simulink model "roundabout_onthego_path"  (R2016b)
settings: Solver=FixedStepAuto  StartTime=0.0  StopTime=inf  RelTol=1e-3
undefined symbols (not defined in the file): DiscIntNeverNeededParam, vehicle_name
libraries: simulink x8, SCANeR_API x6
(part 2 of 2)

== matlab function roundabout_onthego_path/MATLAB Function ==
  data: r input; y output [0..1000]; exit input
function y = fcn(r, exit)

 
r_off = 1.5;
lambda = 10; 
degtorad = pi/180;
center_x = 0; 
center_y = 0;
angle = linspace(0, 2*pi, 360); 
x_circle = r*cos(angle) + center_x; 
y_circle = r*sin(angle) + center_y;
circle_start_angle = 10;
qs_x = r_off; qs_y = -30;
p1_x = center_x + (r+r_off)*cos((lambda-90)*degtorad); 
p1_y = center_y + (r+r_off)*sin((lambda-90)*degtorad);
p2_x = center_x + (r)*cos(-lambda*degtorad);
p2_y = center_y + (r)*sin(-lambda*degtorad);

npts = 8 ;

cl1_theta0 = 90*degtorad; cl1_theta1 = 10*degtorad;
cl2_theta0 = 10*degtorad; cl2_theta1 = 30*degtorad; 

[k1,dk1,L1] = buildClothoid(qs_x, qs_y, cl1_theta0, p1_x, p1_y, cl1_theta1);

XY1 = pointsOnClothoid(qs_x, qs_y, cl1_theta0, k1, dk1, L1, npts) ;
XY4 = zeros(size(XY1,1), size(XY1,2)); XY6 = zeros(size(XY1,1), size(XY1,2));
XY8 = zeros(size(XY1,1), size(XY1,2)); XY10 = zeros(size(XY1,1), size(XY1,2));
XY6(1,:) = XY1(1,:); XY6(2,:)= -XY1(2,:);

XY8(1,:) = XY1(2,:); XY8(2,:)=XY1(1,:);

XY10(1,:) = -XY1(1,:); XY10(2,:)=XY1(2,:);

XY4(1,:) = -XY8(1,:); XY4(2,:) = -XY8(2,:);


%---- sequentialize ----------- %


XY4(1,:) = XY4(1,end:-1:1); XY4(2,:) = XY4(2,end:-1:1);

XY6(1,:) = XY6(1,end:-1:1); XY6(2,:) = XY6(2,end:-1:1);

XY8(1,:) = XY8(1,end:-1:1); XY8(2,:) = XY8(2,end:-1:1);

XY10(1,:) = XY10(1,end:-1:1); XY10(2,:) = XY10(2,end:-1:1);



start_deg = 10; deg_len = (90*exit)-(2*start_deg); npts_arc = (deg_len - (exit*20)); step_size = (deg_len/npts_arc); 
arc1_x = zeros(1,npts_arc);
arc1_y = zeros(1,npts_arc);
for i = 1:npts_arc
    ang = start_deg + i*step_size;
    arc1_x(i) = center_x + (r+r_off)*cos((ang-90)*degtorad);
    arc1_y(i) = center_y + (r+r_off)*sin((ang-90)*degtorad);
end


if exit == 1
    comb_x = [XY1(1,:) arc1_x(1,:) XY4(1,:)];
    comb_y = [XY1(2,:) arc1_y(1,:) XY4(2,:)];
end
if exit == 2
    comb_x = [XY1(1,:) arc1_x(1,:) XY6(1,:)];
    comb_y = [XY1(2,:) arc1_y(1,:) XY6(2,:)];
end
if exit == 3
    comb_x = [XY1(1,:) arc1_x(1,:) XY8(1,:)];
    comb_y = [XY1(2,:) arc1_y(1,:) XY8(2,:)];
end
if exit == 4
    comb_x = [XY1(1,:) arc1_x(1,:) XY10(1,:)];
    comb_y = [XY1(2,:) arc1_y(1,:) XY10(2,:)];
end
plot(comb_x, comb_y);

y = [comb_x', comb_y'];
% y = comb_x; 
end

function [ k, dk, L, iter, varargout ] = buildClothoid( x0, y0, theta0, x1, y1, theta1 )

  dx  = x1 - x0 ;
  dy  = y1 - y0 ;
  r   = sqrt( dx^2 + dy^2 ) ;
  phi = atan2( dy, dx ) ;

  phi0  = normalizeAngle(theta0 - phi) ;
  phi1  = normalizeAngle(theta1 - phi) ;
  delta = phi1 - phi0 ;

  % initial point
  Aguess = guessA( phi0, phi1 ) ;

  % Newton iteration
  [A,iter] = findA( Aguess, delta, phi0, 1e-12 ) ;

  % final operation
  [h,g] = GeneralizedFresnelCS( 1, 2*A, delta-A, phi0 ) ;
  L = r/h ;

  if L > 0
    k  = (delta - A)/L ;
    dk = 2*A/L^2 ;
  else
    error('negative length') ;
  end

  if nargout == 10

    [X,Y] = GeneralizedFresnelCS( 3, 2*A, delta-A, theta0 ) ;
    
    if true
      alpha = X(1)*X(2) + Y(1)*Y(2) ;
      beta  = X(1)*X(3) + Y(1)*Y(3) ;
      gamma = X(1)^2+Y(1)^2 ;
      tx    = X(2)-X(3) ;
      ty    = Y(2)-Y(3) ;
      txy   = L*(X(2)*Y(3)-X(3)*Y(2)) ;
      omega = L*(Y(1)*tx-X(1)*ty) - txy ;
      delta = X(1)*tx + Y(1)*ty ;

      L_1  = omega/delta ; % L_0
      L_2  = txy/delta ; % L_1

      delta = delta * L ;
      k_1  = (beta-gamma-k*omega)/delta ; % k_0
      k_2  = -(beta+k*txy)/delta ; % k_1

      delta = delta * L/2 ;
      dk_1 = (gamma-alpha-dk*omega*L)/delta ; % dk_0    
      dk_2 = (alpha-dk*txy*L)/delta ; % dk_1
    else
      dkL = dk*L ;
      M = [ X(1) - L*(dkL*Y(3)+k*Y(2)), -L*Y(2), -L*Y(3) ; ...
            Y(1) + L*(dkL*X(3)+k*X(2)),  L*X(2),  L*X(3) ; ...
            dkL+k,                            1,       1 ] ;
      tmp = M\[L*Y(1);-L*X(1);-1] ;
      L_1  = tmp(1) ;
      k_1  = tmp(2)/L ;
      dk_1 = 2*tmp(3)/L^2 ;
      tmp = M\[0;0;1] ;
      L_2  = tmp(1) ;
      k_2  = tmp(2)/L ;
      dk_2 = 2*tmp(3)/L^2 ;
    end
    
    varargout{1} = k_1 ; % k_0
    varargout{2} = dk_1 ; % dk_0
    varargout{3} = L_1 ; % L_0
    
    varargout{4} = k_2 ; % k_1
    varargout{5} = dk_2 ; % dk_1
    varargout{6} = L_2 ; % L_1

  elseif nargout > 4
    error('expected <= 4 or 10 output argument') ;
  end 
  
end

%=========================================================================%
%  normalizeAngle:  normalize angle in the range [-pi,pi]                 %
%=========================================================================%
function phi = normalizeAngle( phi_in )
  phi = phi_in ;
  while ( phi > pi )
    phi = phi - 2*pi ;
  end
  while ( phi < -pi )
    phi = phi + 2*pi ;
  end
end

%=========================================================================%
%  findA:  Find a zero of function g(A) defined as                        %
%  g(A) = \int_0^1 \sin( A*t^2+(delta-A)*t+phi0 ) dt                      %
%                                                                         %
%  USAGE:  A = findA( Aguess, delta, phi0, tol );                         %
%                                                                         %
%  Given an initial guess Aguess find the closest zero of equation g(A)   %
%                                                                         %
%  On input:                                                              %
%    Aguess      = initial guess.                                         %
%    delta, phi0 = Angles used in the clothoid fitting problem.           %
%    tol         = Tolerance for stopping criterium of Newton iteration.  %
%                                                                         %
%  On output:                                                             %
%    A           = the zero of function g(A) closest to Aguess.           %
%    iter        = iteration performed                                    %
%                                                                         %
%=========================================================================%
function [A,iter] = findA( Aguess, delta, phi0, tol )
  A = Aguess ;
  for iter=1:100
    [intC,intS] = GeneralizedFresnelCS( 3, 2*A, delta-A, phi0 ) ;
    f  = intS(1) ;
    df = intC(3)-intC(2) ;
    A  = A - f/df ;
    if abs(f) < tol
      break ;
    end
  end
  if abs(f) > tol*10
    fprintf( 1, 'Newton iteration fails, f = %g\n', f ) ;
    fprintf( 1, 'Aguess = %g, A = %g, delta = %g , phi0 = %g\n', Aguess, A, delta, phi0 ) ;
  end
end

%=========================================================================%
%  guessA:  Find guess for zeros of function g(A)                         %
%                                                                         %
%  USAGE:  A = guessA( phi0, phi1 );                                      %
%                                                                         %
%  On input:                                                              %
%       phi0, phi1 = Angles used in the clothoid fitting problem.         %
%                                                                         %
%  On output:                                                             %
%       A = an approximate zero of function g(A).                         %
%                                                                         %
%=========================================================================%
function A = guessA( phi0, phi1 )
  CF = [ 2.989696028701907, ...
         0.716228953608281, ...
        -0.458969738821509, ...
        -0.502821153340377, ...
         0.261062141752652, ...
        -0.045854475238709 ] ;
  X  = phi0/pi ;
  Y  = phi1/pi ;
  xy = X*Y ;
  A  = (phi0+phi1) * ( CF(1) + xy * ( CF(2) + xy * CF(3) ) + ...
                       (CF(4) + xy * CF(5)) * (X^2+Y^2) + ...
                        CF(6) * (X^4+Y^4) ) ;
end

function varargout = pointsOnClothoid( varargin )
  
  if nargin == 2
    if isstruct(varargin{1})
      x0     = varargin{1}.x0 ;
      y0     = varargin{1}.y0 ;
      theta0 = varargin{1}.theta0 ;
      kappa  = varargin{1}.kappa ;
      dkappa = varargin{1}.dkappa ;
      L      = varargin{1}.L ;
      npts   = varargin{2} ;
      tvec   = [0:L/(npts-1):L] ;
    else
      error('expexted struct as first arument') ;
    end
  elseif nargin == 6 || nargin == 7
    x0     = varargin{1} ;
    y0     = varargin{2} ;
    theta0 = varargin{3} ;
    kappa  = varargin{4} ;
    dkappa = varargin{5} ;
    L      = varargin{6} ;
    if nargin == 7
      npts = varargin{7} ;
      tvec = [0:L/(npts-1):L] ;
    else
      tvec = L ;
    end
  else
    error('expexted 2,6 or 7 input arguments') ;
  end
  
  X = [] ;
  Y = [] ;
  for t=tvec(1,1):tvec(1,end)
    [C,S] = GeneralizedFresnelCS( 1, dkappa*t^2, kappa*t, theta0 ) ;
    X = [ X x0 + t*C ] ;
    Y = [ Y y0 + t*S ] ;
  end
  if nargout > 1
    varargout{1} = X ;
    varargout{2} = Y ;
  else
    varargout{1} = [X ; Y] ;
  end
end

function [X,Y] = GeneralizedFresnelCS( nk, a, b, c )

  epsi = 1e-2 ; % best thresold

  if abs(a) < epsi % case `a` small
    [X,Y] = evalXYaSmall( nk, a, b, 3 ) ;
  else
    [X,Y] = evalXYaLarge( nk, a, b ) ;
  end

  cc = cos(c) ;
  ss = sin(c) ;

  for k=1:nk
    xx = X(k) ;
    yy = Y(k) ;
    X(k) = xx*cc-yy*ss ;
    Y(k) = xx*ss+yy*cc ;
  end

end
%
%
%
function [C,S] = FresnelCSk( nk, t )
  C = zeros(nk,1) ;
  S = zeros(nk,1) ;
  [C(1),S(1)] = FresnelCS(t) ;
  if nk > 1
    tt   = pi/2*t^2 ;
    ss   = sin(tt) ;
    cc   = cos(tt) ;
    C(2) = ss/pi ;
    S(2) = (1-cc)/pi ;
    if nk > 2
      C(3) = (t*ss-S(1))/pi ;
      S(3) = (C(1)-t*cc)/pi ;
    end
  end
end
%
%
%
function [X,Y] = evalXYaLarge( nk, a, b )
  X       = zeros(nk,1) ;
  Y       = zeros(nk,1) ;
  s       = sign(a) ;
  z       = sqrt(abs(a)/pi) ;
  ell     = s*b/sqrt(abs(a)*pi) ;
  g       = -0.5*s*b^2/abs(a) ;
  [Cl,Sl] = FresnelCSk(nk,ell) ;
  [Cz,Sz] = FresnelCSk(nk,ell+z) ;
  dC      = Cz - Cl ;
  dS      = Sz - Sl ;
  cg      = cos(g)/z ;
  sg      = sin(g)/z ;
  X(1)    = cg * dC(1) - s * sg * dS(1) ;
  Y(1)    = sg * dC(1) + s * cg * dS(1) ;
  if nk > 1
    cg   = cg/z ;
    sg   = sg/z ;
    DC   = dC(2)-ell*dC(1);
    DS   = dS(2)-ell*dS(1);
    X(2) = cg * DC - s * sg * DS ;
    Y(2) = sg * DC + s * cg * DS ;
    if nk > 2
      cg   = cg/z ;
      sg   = sg/z ;
      DC   = dC(3)+ell*(ell*dC(1)-2*dC(2)) ;
      DS   = dS(3)+ell*(ell*dS(1)-2*dS(2)) ;
      X(3) = cg * DC - s * sg * DS ;
      Y(3) = sg * DC + s * cg * DS ;
    end
  end
end
%
%
%
function res = rLommel_MATLAB(mu, nu, z)
  a   = mu-nu+1 ;
  b   = mu+nu+1 ;
  res = eval(hypergeom(1,[a/2+1,b/2+1],-z^2/4)/(a*b)) ;
end
%
%
%
function res = rLommel(mu,nu,b)
  tmp = 1/((mu+nu+1)*(mu-nu+1)) ;
  res = tmp ;
  for n=1:100
    tmp = tmp * (-b/(2*n+mu-nu+1)) * (b/(2*n+mu+nu+1)) ;
    res = res + tmp ;
    if abs(tmp) < abs(res) * 1e-50
      break ;
    end;
  end
end
%
%
%
function [X,Y] = evalXYazero( nk, b )
  X  = zeros(nk,1) ;
  Y  = zeros(nk,1) ;
  sb = sin(b);
  cb = cos(b);
  b2 = b*b ;
  if abs(b) < 1e-3
    X(1) = 1-(b2/6)*(1-(b2/20)*(1-(b2/42))) ;
    Y(1) = (b/2)*(1-(b2/12)*(1-(b2/30))) ;
  else
    X(1) = sb/b ;
    Y(1) = (1-cb)/b ;
  end
  % use recurrence in the stable part
  m = min( [ max([1,floor(2*b)]), nk] ) ;
  for k=1:m-1
    X(k+1) = (sb-k*Y(k))/b ;
    Y(k+1) = (k*X(k)-cb)/b ;
  end
  % use Lommel for the unstable part
  if m < nk
    A   = b*sb ;
    D   = sb-b*cb ;
    B   = b*D ;
    C   = -b2*sb ;
    rLa = rLommel(m+1/2,3/2,b) ;
    rLd = rLommel(m+1/2,1/2,b) ;
    for k=m:nk-1
      rLb    = rLommel(k+3/2,1/2,b) ;
      rLc    = rLommel(k+3/2,3/2,b) ;
      X(k+1) = ( k*A*rLa + B*rLb + cb )/(1+k) ;
      Y(k+1) = ( C*rLc + sb ) / (2+k) + D*rLd ;
      rLa = rLc ;
      rLd = rLb ;
    end
  end
end
%
%
%
function [X,Y] = evalXYaSmall( nk, a, b, p )
  [X0,Y0] = evalXYazero( nk + 4*p + 2, b ) ;

  X    = zeros(nk,1) ;
  Y    = zeros(nk,1) ;
  tmpX = zeros(p+1,1) ;
  tmpY = zeros(p+1,1) ;

  for j=1:nk
    tmpX(1) = X0(j)-(a/2)*Y0(j+2) ;
    tmpY(1) = Y0(j)+(a/2)*X0(j+2) ;
    t  = 1 ;
    aa = -(a/2)^2 ;
    for n=1:p
      ii = 4*n+j ;
      t  = t*(aa/(2*n*(2*n-1))) ;
      bf = a/(4*n+2) ;
      tmpX(1+n) = t*(X0(ii)-bf*Y0(ii+2)) ;
      tmpY(1+n) = t*(Y0(ii)+bf*X0(ii+2)) ;
    end
    X(j) = sum(tmpX) ;
    Y(j) = sum(tmpY) ;
  end
end

function [FresnelC,FresnelS] = FresnelCS(y)
%******************************************************************************
% FresnelCS:  Compute Fresnel sine and cosine integrals                       %
%                                                                             %
% USAGE: [FresnelC,FresnelS] = FresnelCS(y) ;                                 %
%                                                                             %
%  Fresnel integral are defined as:                                           %
%                                                                             %
%  C(y) = \int_0^y cos( (pi/2)*t^2 ) dt                                       %
%  S(y) = \int_0^y sin( (pi/2)*t^2 ) dt                                       %
%                                                                             %
% The algorithm is described in:                                              %
%   Atlas for computing mathematical functions : an illustrated guide for     %
%   practitioners, with programs in C and Mathematica / William J. Thompson.  %
%   New York : Wiley, c1997.                                                  %
%                                                                             %
% The cose is a sligly modification of original code developed by             %
% Venkata Sivakanth Telasula (sivakanth.telasula@gmail.com)                   %
%                                                                             %
% On input:                                                                   %
%                                                                             %
%       y = argument of the function C(y) and S(y), it may be a vector        %
%                                                                             %
% On output:                                                                  %
%                                                                             %
%       FresnelC = The value(s) of C(y)                                       %
%       FresnelS = The value(s) of S(y)                                       %
%                                                                             %
%******************************************************************************

  fn = [ 0.49999988085884732562,   ...
         1.3511177791210715095,    ...
         1.3175407836168659241,    ...
         1.1861149300293854992,    ...
         0.7709627298888346769,    ...
         0.4173874338787963957,    ...
         0.19044202705272903923,   ...
         0.06655998896627697537,   ...
         0.022789258616785717418,  ...
         0.0040116689358507943804, ...
         0.0012192036851249883877 ] ;
  
  fd = [ 1.0,                      ...
         2.7022305772400260215,    ...
         4.2059268151438492767,    ...
         4.5221882840107715516,    ...
         3.7240352281630359588,    ...
         2.4589286254678152943,    ...
         1.3125491629443702962,    ...
         0.5997685720120932908,    ...
         0.20907680750378849485,   ...
         0.07159621634657901433,   ...
         0.012602969513793714191,  ...
         0.0038302423512931250065 ] ;
  
  gn = [ 0.50000014392706344801,    ...
         0.032346434925349128728,   ...
         0.17619325157863254363,    ...
         0.038606273170706486252,   ...
         0.023693692309257725361,   ...
         0.007092018516845033662,   ...
         0.0012492123212412087428,  ...
         0.00044023040894778468486, ...
        -8.80266827476172521e-6,    ...
        -1.4033554916580018648e-8,  ...
        2.3509221782155474353e-10 ] ;
  
  gd  = [ 1.0,                      ...
          2.0646987497019598937,    ...
          2.9109311766948031235,    ...
          2.6561936751333032911,    ...
          2.0195563983177268073,    ...
          1.1167891129189363902,    ...
          0.57267874755973172715,   ...
          0.19408481169593070798,   ...
          0.07634808341431248904,   ...
          0.011573247407207865977,  ...
          0.0044099273693067311209, ...
         -0.00009070958410429993314 ] ;

  FresnelC = zeros(size(y));
  FresnelS = zeros(size(y));
  
  for j = 1:length(y)
    x = abs(y(j)) ;
    if x < 1.0
      t = -((pi/2)*x.^2).^2;
      % Cosine integral series
      twofn   = 0.0 ;
      fact    = 1.0 ;
      denterm = 1.0 ;
      numterm = 1.0 ;
      sum     = 1.0 ;
      ratio   = 10.0 ; 
 
      while ratio > eps
        twofn   = twofn + 2.0;
        fact    = fact*twofn*(twofn-1.0);
        denterm = denterm + 4.0;
        numterm = numterm*t;
        term    = numterm/(fact*denterm);
        sum     = sum+term;
        ratio   = abs(term/sum);
      end

      FresnelC(j) = x*sum;
 
      % Sine integral series
      twofn   = 1.0 ;
      fact    = 1.0 ;
      denterm = 3.0 ;
      numterm = 1.0 ;
      sum     = 1.0/3.0 ;
      ratio   = 10.0 ;
 
      while ratio > eps
        twofn   = twofn+2.0;
        fact    = fact*twofn*(twofn-1.0);
        denterm = denterm+4.0;
        numterm = numterm*t;
        term    = numterm/(fact*denterm);
        sum     = sum+term;
        ratio   = abs(term/sum);
      end
 
      FresnelS(j) = (pi/2)*sum.*x.^3;

    elseif x < 6.0

      % Rational approximation for f
      sumn = 0.0 ;
      sumd = fd(12) ;
      for k=11:-1:1
        sumn = fn(k)+x*sumn ;
        sumd = fd(k)+x*sumd ;
      end
      f = sumn/sumd;
      % Rational approximation for  g
      sumn = 0.0 ;
      sumd = gd(12) ;
      for k=11:-1:1
        sumn = gn(k)+x*sumn;
        sumd = gd(k)+x*sumd;
      end
      g    = sumn/sumd;
      U    = (pi/2)*x.^2 ;
      SinU = sin(U);
      CosU = cos(U);
      FresnelC(j) = 0.5+f*SinU-g*CosU;
      FresnelS(j) = 0.5-f*CosU-g*SinU;
    else
      % x >= 6; asymptotic expansions for  f  and  g
      t = -(pi*x.^2)^(-2.0) ;
      % Expansion for  f
      numterm = -1.0 ;
      term    =  1.0 ;
      sum     =  1.0 ;
      oldterm =  1.0 ;
      ratio   = 10.0 ;
      eps10   = 0.1*eps;

      while ratio > eps10
        numterm = numterm+4.0;
        term    = term*numterm*(numterm-2.0)*t;
        sum     = sum + term;
        absterm = abs(term);
        ratio   = abs(term/sum);
        if oldterm < absterm
          disp('\n\n !!In FresnelCS f not converged to eps');
          ratio = eps10;
        end
        oldterm = absterm;
      end

      f = sum/(pi*x);
      % Expansion for  g
      numterm = -1.0 ;
      term    =  1.0 ;
      sum     =  1.0 ;
      oldterm =  1.0 ; 
      ratio   = 10.0 ;
      eps10   = 0.1*eps ;

      while ratio > eps10
        numterm = numterm+ 4.0;
        term    = term*numterm*(numterm+2.0)*t;
        sum     = sum+term;
        absterm = abs(term);
        ratio   = abs(term/sum);
        if oldterm < absterm
          disp('\n\n!!In FresnelCS g not converged to eps');
          ratio = eps10;
        end
        oldterm = absterm;
      end
      g    = sum/((pi*x)^2*x) ;
      U    = (pi/2)*x.^2 ;
      SinU = sin(U);
      CosU = cos(U);
      FresnelC(j) = 0.5+f*SinU-g*CosU;
      FresnelS(j) = 0.5-f*CosU-g*SinU;
    end
    if y(j) < 0
      FresnelC(j) = -FresnelC(j) ;
      FresnelS(j) = -FresnelS(j) ;
    end
  end
end
% EOF

== stateflow chart roundabout_onthego_path/Subsystem/Chart1 ==
  state Speed_Control/
    state Control_Off/
      accel = 0;
      brake = 0;
      int_epsilon = 0;
      Gear=3;
    state Controller/
      limit_accel = 1/kp_acc;
      limit_brake = 1/kp_brk;
      state normal_regulation/
        state normal_accel/
          control_state = 2;
          accel = -kp_acc*epsilon - ki_acc*int_epsilon;
          brake = 0;
          Gear_d = Gear;
        state normal_brake/
          control_state = 1;
          brake = kp_brk*epsilon + ki_brk*int_epsilon;
          accel = 0;
          Gear_d = Gear;
        (junction 58) -> (junction 59) [order 1] : [epsilon <= tolerance]
        (junction 58) -> (junction 57) [order 2]
        (junction 59) -> Speed_Control.Controller.normal_regulation.normal_accel [order 1] : [abs(epsilon) < limit_accel & control_state == 2]
            | {int_epsilon = int_epsilon + step_size*epsilon;}
        (junction 59) -> Speed_Control.Controller.normal_regulation.normal_accel [order 2] : {int_epsilon = 0;}
        (junction 57) -> Speed_Control.Controller.normal_regulation.normal_brake [order 1] : [abs(epsilon) < limit_brake & control_state == 1]
            | {int_epsilon = int_epsilon + step_size*epsilon;}
        (junction 57) -> Speed_Control.Controller.normal_regulation.normal_brake [order 2] : {int_epsilon = 0;}
        Speed_Control.Controller.normal_regulation.normal_brake -> (junction 69)
        Speed_Control.Controller.normal_regulation.normal_accel -> (junction 69)
      state reverse_regulation1/
        state normal_accel/
          control_state = 2;
          accel = -kp_acc*epsilon - ki_acc*int_epsilon;
          brake = 0;
          Gear_d = Gear;
        state normal_brake/
          control_state = 1;
          brake = kp_brk*epsilon + ki_brk*int_epsilon;
          accel = 0;
          Gear_d = Gear;
        (junction 123) -> (junction 124) [order 1] : [epsilon <=-0.1]
        (junction 123) -> (junction 125) [order 2]
        (junction 124) -> Speed_Control.Controller.reverse_regulation1.normal_accel [order 1] : [abs(epsilon) < limit_accel & control_state == 2]
            | {int_epsilon = int_epsilon + step_size*epsilon;}
        (junction 124) -> Speed_Control.Controller.reverse_regulation1.normal_accel [order 2] : {int_epsilon = 0;}
        (junction 125) -> Speed_Control.Controller.reverse_regulation1.normal_brake [order 1] : [abs(epsilon) < limit_brake & control_state == 1]
            | {int_epsilon = int_epsilon + step_size*epsilon;}
        (junction 125) -> Speed_Control.Controller.reverse_regulation1.normal_brake [order 2] : {int_epsilon = 0;}
        Speed_Control.Controller.reverse_regulation1.normal_brake -> (junction 126)
        Speed_Control.Controller.reverse_regulation1.normal_accel -> (junction 126)
      (junction 56) -> (junction 99) [order 1] : [setpoint< 0]
          | {epsilon =- speed+setpoint;}
      (junction 56) -> (junction 62) [order 2] : {epsilon = speed-setpoint;}
      (junction 62) -> (junction 58) : {Gear =10;}
      (junction 69) -> (junction 56)
      (junction 126) -> (junction 56)
      (junction 99) -> (junction 123) : {Gear =2;}
    (default) -> (junction 55)
    (junction 55) -> Control_Off [order 1] : [speed_control_on == 0]
    Control_Off -> (junction 55)
    Controller -> (junction 55) : [speed_control_on == 0]
    (junction 55) -> (junction 56) [order 2] : {control_state = 0;}
  data: speed input double; setpoint input double; speed_control_on input double; accel output double; brake output double; kp_acc input double; ki_acc input double; kp_brk input double; ki_brk input double; step_size input double; limit_accel local double; limit_brake local double; epsilon output double; int_epsilon output double; control_state output double; Gear_d output double; Gear local double; tolerance input double

== matlab function roundabout_onthego_path/Subsystem/MATLAB Function ==
  data: vehicle_name input; Kp_Accl output; Ki_Accl output; Intended_Vehicle_Speed_kmph input
function [Kp_Accl, Ki_Accl]= fcn(vehicle_name,Intended_Vehicle_Speed_kmph)
% This function calculates the Kp_Accl and Ki_Accl
% Following are the vehicle models to be used for simulation
% Vehicle_name:
% 0 = HHN
% 1 = BCB
% 2 = FFK
% 3 = KFKL1
% 4 = KFKL2
% 5 = KFKL1_VODM_CD04
% 6= KFKL1_VODM_CD05
% 7 = KFKL1_VODM_CD06
% 8 = FFKL1_VODM_CD06
% 9 = FFKL1_MMAC_CD06
% 10 = FFKL2_MMAC_CD06
% 11 = KFKL2_MMAC_CD06
% 12 = XDD

if (vehicle_name == 0)
    Kp_Accl = 0.3;
    Ki_Accl = 0.05;
elseif (vehicle_name == 1)
    Kp_Accl = 0.3;
    Ki_Accl = 0.05;
elseif (vehicle_name == 2)
    Kp_Accl = 0.1;
    Ki_Accl = 0.02;
elseif (vehicle_name == 3)
    Kp_Accl = 0.3;
    Ki_Accl = 0.02;
elseif (vehicle_name == 4)
    Kp_Accl = 0.3;
    Ki_Accl = 0.02;
elseif (vehicle_name == 5)
    Kp_Accl = 0.3;
    Ki_Accl = 0.02;
elseif (vehicle_name == 6)
    Kp_Accl = 0.3;
    Ki_Accl = 0.02;
elseif (vehicle_name == 7)
    Kp_Accl = 0.3;
    Ki_Accl = 0.02;
elseif (vehicle_name == 8)
    Kp_Accl = 0.3;
    Ki_Accl = 0.02;
elseif (vehicle_name == 9)
    Kp_Accl = 0.3;
    Ki_Accl = 0.02;
elseif (vehicle_name == 10)
    Kp_Accl = 0.3;
    Ki_Accl = 0.02;
elseif (vehicle_name == 11)
    Kp_Accl = 0.3;
    Ki_Accl = 0.02;
elseif (vehicle_name == 17)% HCB 60kwh
    if Intended_Vehicle_Speed_kmph >= 60
        Kp_Accl = 0.3; %0.1
        Ki_Accl = 0.05;%0.01
    else
        Kp_Accl = 0.1; %0.1
        Ki_Accl = 0.01;%0.01
    end
elseif (vehicle_name == 13) || (vehicle_name == 15) % BCB
    Kp_Accl =0.3;
    Ki_Accl = 0.05;
elseif (vehicle_name == 18) || (vehicle_name == 14) || (vehicle_name == 12)% XDD vehicle
    Kp_Accl = 0.3;
    Ki_Accl = 0.05;
elseif (vehicle_name == 19)% BCB 40kwh Correl
    if Intended_Vehicle_Speed_kmph >= 50
        Kp_Accl = 1;
        Ki_Accl = 0.1;
    else
        Kp_Accl = 0.1; %0.1
        Ki_Accl = 0.01;%0.01
    end
elseif (vehicle_name == 16) % HHN Correl
    if Intended_Vehicle_Speed_kmph >= 15
        Kp_Accl = 0.3;
        Ki_Accl = 0.05;
    elseif Intended_Vehicle_Speed_kmph < 7
        Kp_Accl = 0.3;
        Ki_Accl = 0.05;
    else
        Kp_Accl = 0.009;
        Ki_Accl = 0.00032;
    end
elseif (vehicle_name == 20) % Echo
    Kp_Accl = 0.3;
    Ki_Accl = 0.05;
elseif (vehicle_name == 21) % Torque Management
    Kp_Accl = 0.0012;
    Ki_Accl = 0.0012;
else  % Other vehicles
    if Intended_Vehicle_Speed_kmph >= 15
        Kp_Accl = 0.3;
        Ki_Accl = 0.05;
    else
        Kp_Accl = 0.009;
        Ki_Accl = 0.00032;
    end
end
